simulink library "ESTS_VHSO"  (R2024b)
settings: Solver=VariableStepAuto  StartTime=0.0  StopTime=10.0  RelTol=1e-3
undefined symbols (not defined in the file or in its folder): ESTS_HVSO_p_SwtRefSped_na, p_RatGearFr_na, p_RatGearRe_na
libraries: ESTS_BRK x1, ESTS_LNGSL x1, ESTS_RBA x1, ESTS_REV x1, ESTS_RSL x1, ESTS_SLA x1, ESTS_TFX x1, ESTS_VSLARE x1, ESTS_TFY x1
settings Model: Creator=blatak  LastModifiedBy=blatak
settings ModelReferenceCC: EnableRefExpFcnMdlSchedulingChecks=on
settings RTWCC: GPUComputeCapability=3.5

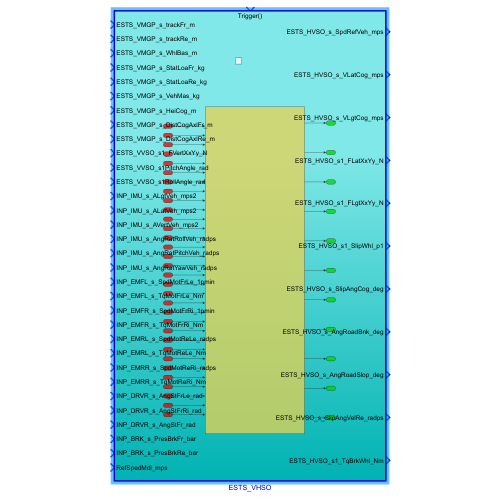
[thumbnail: Simulink's stored preview of the top-level diagram]
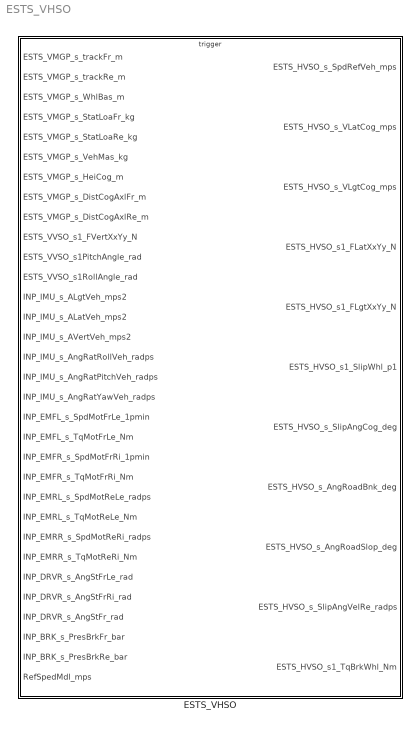
== system ESTS_VHSO ==
  ESTS_VHSO : Subsystem  Description=Horizontal vehicle observer

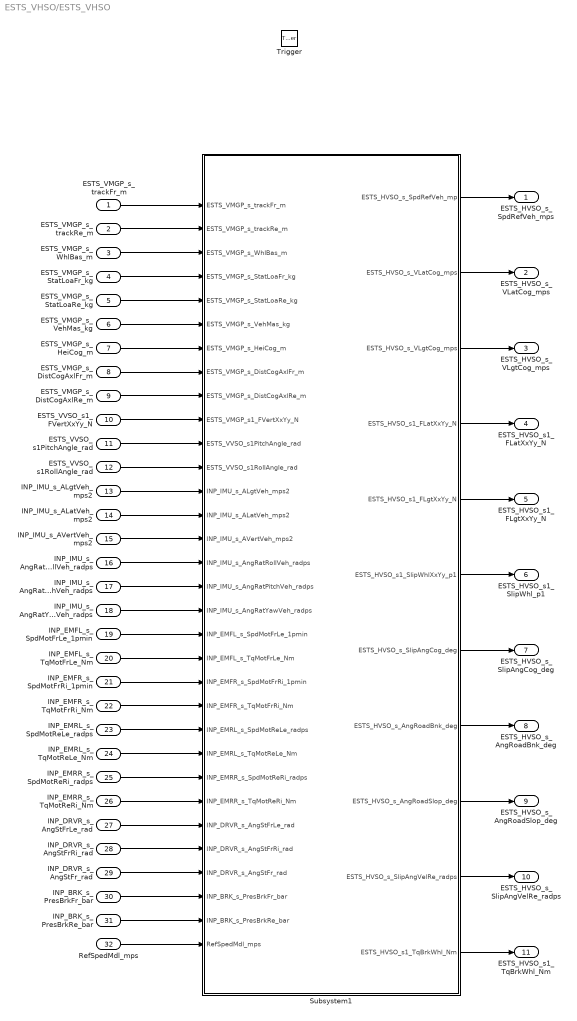
== system ESTS_VHSO/ESTS_VHSO ==
  ESTS_VMGP_s_trackFr_m : Inport
  ESTS_VMGP_s_trackRe_m : Inport  Port=2
  ESTS_VMGP_s_WhlBas_m : Inport  Port=3
  ESTS_VMGP_s_StatLoaFr_kg : Inport  Port=4
  ESTS_VMGP_s_StatLoaRe_kg : Inport  Port=5
  ESTS_VMGP_s_VehMas_kg : Inport  Port=6
  ESTS_VMGP_s_HeiCog_m : Inport  Port=7
  ESTS_VMGP_s_DistCogAxlFr_m : Inport  Port=8
  ESTS_VMGP_s_DistCogAxlRe_m : Inport  Port=9
  ESTS_VVSO_s1_FVertXxYy_N : Inport  Port=10
  ESTS_VVSO_s1PitchAngle_rad : Inport  Port=11
  ESTS_VVSO_s1RollAngle_rad : Inport  Port=12
  INP_IMU_s_ALgtVeh_mps2 : Inport  Port=13
  INP_IMU_s_ALatVeh_mps2 : Inport  Port=14
  INP_IMU_s_AVertVeh_mps2 : Inport  Port=15
  INP_IMU_s_AngRatRollVeh_radps : Inport  Port=16
  INP_IMU_s_AngRatPitchVeh_radps : Inport  Port=17
  INP_IMU_s_AngRatYawVeh_radps : Inport  Port=18
  INP_EMFL_s_SpdMotFrLe_1pmin : Inport  Port=19
  INP_EMFL_s_TqMotFrLe_Nm : Inport  Port=20
  INP_EMFR_s_SpdMotFrRi_1pmin : Inport  Port=21
  INP_EMFR_s_TqMotFrRi_Nm : Inport  Port=22
  INP_EMRL_s_SpdMotReLe_radps : Inport  Port=23
  INP_EMRL_s_TqMotReLe_Nm : Inport  Port=24
  INP_EMRR_s_SpdMotReRi_radps : Inport  Port=25
  INP_EMRR_s_TqMotReRi_Nm : Inport  Port=26
  INP_DRVR_s_AngStFrLe_rad : Inport  Port=27
  INP_DRVR_s_AngStFrRi_rad : Inport  Port=28
  INP_DRVR_s_AngStFr_rad : Inport  Port=29
  INP_BRK_s_PresBrkFr_bar : Inport  Port=30
  INP_BRK_s_PresBrkRe_bar : Inport  Port=31
  RefSpedMdl_mps : Inport  Port=32
  Trigger : TriggerPort  TriggerType=function-call  VariantControl=(inherit)  PortDimensions=1
  Subsystem1 : Subsystem
  ESTS_HVSO_s_SpdRefVeh_mps : Outport
  ESTS_HVSO_s_VLatCog_mps : Outport  Port=2
  ESTS_HVSO_s_VLgtCog_mps : Outport  Port=3
  ESTS_HVSO_s1_FLatXxYy_N : Outport  Port=4
  ESTS_HVSO_s1_FLgtXxYy_N : Outport  Port=5
  ESTS_HVSO_s1_SlipWhl_p1 : Outport  Port=6
  ESTS_HVSO_s_SlipAngCog_deg : Outport  Port=7
  ESTS_HVSO_s_AngRoadBnk_deg : Outport  Port=8
  ESTS_HVSO_s_AngRoadSlop_deg : Outport  Port=9
  ESTS_HVSO_s_SlipAngVelRe_radps : Outport  Port=10
  ESTS_HVSO_s1_TqBrkWhl_Nm : Outport  Port=11
  wires:
  ESTS_VMGP_s_StatLoaFr_kg/1 -> Subsystem1/4(ESTS_VMGP_s_StatLoaFr_kg)
  ESTS_VMGP_s_WhlBas_m/1 -> Subsystem1/3(ESTS_VMGP_s_WhlBas_m)
  ESTS_VMGP_s_trackRe_m/1 -> Subsystem1/2(ESTS_VMGP_s_trackRe_m)
  ESTS_VMGP_s_trackFr_m/1 -> Subsystem1/1(ESTS_VMGP_s_trackFr_m)
  Subsystem1/1(ESTS_HVSO_s_SpdRefVeh_mp) -> ESTS_HVSO_s_SpdRefVeh_mps/1
  Subsystem1/2(ESTS_HVSO_s_VLatCog_mps) -> ESTS_HVSO_s_VLatCog_mps/1
  Subsystem1/3(ESTS_HVSO_s_VLgtCog_mps) -> ESTS_HVSO_s_VLgtCog_mps/1
  Subsystem1/4(ESTS_HVSO_s1_FLatXxYy_N) -> ESTS_HVSO_s1_FLatXxYy_N/1
  Subsystem1/5(ESTS_HVSO_s1_FLgtXxYy_N) -> ESTS_HVSO_s1_FLgtXxYy_N/1
  Subsystem1/6(ESTS_HVSO_s1_SlipWhlXxYy_p1) -> ESTS_HVSO_s1_SlipWhl_p1/1
  Subsystem1/7(ESTS_HVSO_s_SlipAngCog_deg) -> ESTS_HVSO_s_SlipAngCog_deg/1
  Subsystem1/8(ESTS_HVSO_s_AngRoadBnk_deg) -> ESTS_HVSO_s_AngRoadBnk_deg/1
  Subsystem1/9(ESTS_HVSO_s_AngRoadSlop_deg) -> ESTS_HVSO_s_AngRoadSlop_deg/1
  ESTS_VMGP_s_StatLoaRe_kg/1 -> Subsystem1/5(ESTS_VMGP_s_StatLoaRe_kg)
  ESTS_VMGP_s_VehMas_kg/1 -> Subsystem1/6(ESTS_VMGP_s_VehMas_kg)
  ESTS_VMGP_s_HeiCog_m/1 -> Subsystem1/7(ESTS_VMGP_s_HeiCog_m)
  ESTS_VVSO_s1_FVertXxYy_N/1 -> Subsystem1/10(ESTS_VMGP_s1_FVertXxYy_N)
  ESTS_VVSO_s1PitchAngle_rad/1 -> Subsystem1/11(ESTS_VVSO_s1PitchAngle_rad)
  ESTS_VVSO_s1RollAngle_rad/1 -> Subsystem1/12(ESTS_VVSO_s1RollAngle_rad)
  INP_IMU_s_ALgtVeh_mps2/1 -> Subsystem1/13(INP_IMU_s_ALgtVeh_mps2)
  INP_IMU_s_AngRatYawVeh_radps/1 -> Subsystem1/18(INP_IMU_s_AngRatYawVeh_radps)
  INP_IMU_s_AngRatPitchVeh_radps/1 -> Subsystem1/17(INP_IMU_s_AngRatPitchVeh_radps)
  INP_IMU_s_AngRatRollVeh_radps/1 -> Subsystem1/16(INP_IMU_s_AngRatRollVeh_radps)
  INP_IMU_s_AVertVeh_mps2/1 -> Subsystem1/15(INP_IMU_s_AVertVeh_mps2)
  INP_IMU_s_ALatVeh_mps2/1 -> Subsystem1/14(INP_IMU_s_ALatVeh_mps2)
  Subsystem1/10(ESTS_HVSO_s_SlipAngVelRe_radps) -> ESTS_HVSO_s_SlipAngVelRe_radps/1
  INP_EMFL_s_SpdMotFrLe_1pmin/1 -> Subsystem1/19(INP_EMFL_s_SpdMotFrLe_1pmin)
  INP_EMFL_s_TqMotFrLe_Nm/1 -> Subsystem1/20(INP_EMFL_s_TqMotFrLe_Nm)
  INP_EMFR_s_SpdMotFrRi_1pmin/1 -> Subsystem1/21(INP_EMFR_s_SpdMotFrRi_1pmin)
  INP_EMFR_s_TqMotFrRi_Nm/1 -> Subsystem1/22(INP_EMFR_s_TqMotFrRi_Nm)
  INP_EMRL_s_SpdMotReLe_radps/1 -> Subsystem1/23(INP_EMRL_s_SpdMotReLe_radps)
  INP_EMRL_s_TqMotReLe_Nm/1 -> Subsystem1/24(INP_EMRL_s_TqMotReLe_Nm)
  INP_EMRR_s_SpdMotReRi_radps/1 -> Subsystem1/25(INP_EMRR_s_SpdMotReRi_radps)
  INP_EMRR_s_TqMotReRi_Nm/1 -> Subsystem1/26(INP_EMRR_s_TqMotReRi_Nm)
  ESTS_VMGP_s_DistCogAxlFr_m/1 -> Subsystem1/8(ESTS_VMGP_s_DistCogAxlFr_m)
  ESTS_VMGP_s_DistCogAxlRe_m/1 -> Subsystem1/9(ESTS_VMGP_s_DistCogAxlRe_m)
  INP_DRVR_s_AngStFrLe_rad/1 -> Subsystem1/27(INP_DRVR_s_AngStFrLe_rad)
  INP_DRVR_s_AngStFrRi_rad/1 -> Subsystem1/28(INP_DRVR_s_AngStFrRi_rad)
  INP_DRVR_s_AngStFr_rad/1 -> Subsystem1/29(INP_DRVR_s_AngStFr_rad)
  RefSpedMdl_mps/1 -> Subsystem1/32(RefSpedMdl_mps)
  INP_BRK_s_PresBrkFr_bar/1 -> Subsystem1/30(INP_BRK_s_PresBrkFr_bar)
  INP_BRK_s_PresBrkRe_bar/1 -> Subsystem1/31(INP_BRK_s_PresBrkRe_bar)
  Subsystem1/11(ESTS_HVSO_s1_TqBrkWhl_Nm) -> ESTS_HVSO_s1_TqBrkWhl_Nm/1

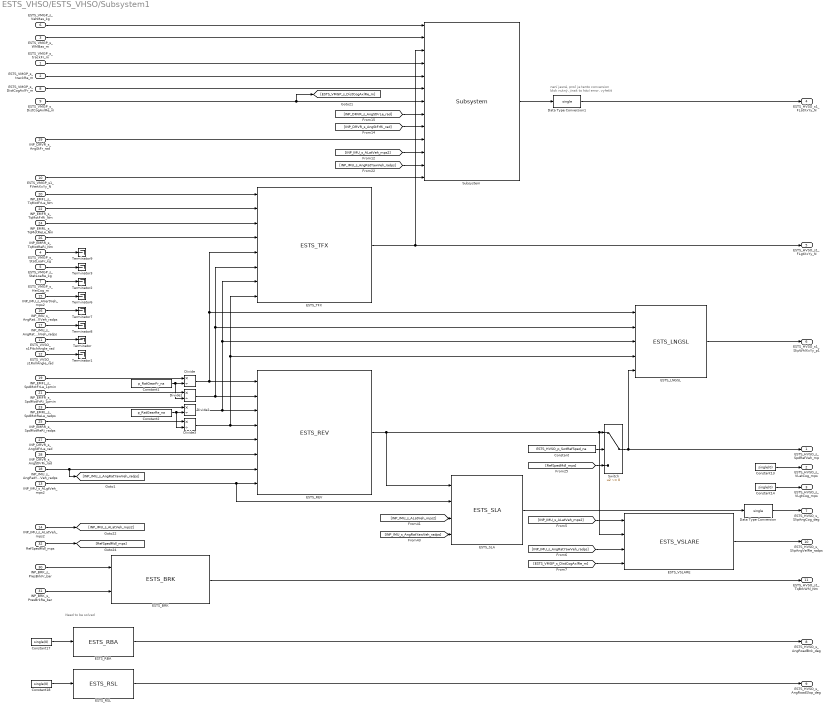
== system ESTS_VHSO/ESTS_VHSO/Subsystem1 ==
  note: není jasné, proč je tento conversion
      | blok nutný, jinak to hází error, vyřešit
  note: Need to be solved
  ESTS_VMGP_s_trackFr_m : Inport
  ESTS_VMGP_s_trackRe_m : Inport  Port=2
  ESTS_VMGP_s_WhlBas_m : Inport  Port=3
  ESTS_VMGP_s_StatLoaFr_kg : Inport  Port=4
  ESTS_VMGP_s_StatLoaRe_kg : Inport  Port=5
  ESTS_VMGP_s_VehMas_kg : Inport  Port=6
  ESTS_VMGP_s_HeiCog_m : Inport  Port=7
  ESTS_VMGP_s_DistCogAxlFr_m : Inport  Port=8
  ESTS_VMGP_s_DistCogAxlRe_m : Inport  Port=9
  ESTS_VMGP_s1_FVertXxYy_N : Inport  Port=10
  ESTS_VVSO_s1PitchAngle_rad : Inport  Port=11
  ESTS_VVSO_s1RollAngle_rad : Inport  Port=12
  INP_IMU_s_ALgtVeh_mps2 : Inport  Port=13
  INP_IMU_s_ALatVeh_mps2 : Inport  Port=14
  INP_IMU_s_AVertVeh_mps2 : Inport  Port=15
  INP_IMU_s_AngRatRollVeh_radps : Inport  Port=16
  INP_IMU_s_AngRatPitchVeh_radps : Inport  Port=17
  INP_IMU_s_AngRatYawVeh_radps : Inport  Port=18
  INP_EMFL_s_SpdMotFrLe_1pmin : Inport  Port=19
  INP_EMFL_s_TqMotFrLe_Nm : Inport  Port=20
  INP_EMFR_s_SpdMotFrRi_1pmin : Inport  Port=21
  INP_EMFR_s_TqMotFrRi_Nm : Inport  Port=22
  INP_EMRL_s_SpdMotReLe_radps : Inport  Port=23
  INP_EMRL_s_TqMotReLe_Nm : Inport  Port=24
  INP_EMRR_s_SpdMotReRi_radps : Inport  Port=25
  INP_EMRR_s_TqMotReRi_Nm : Inport  Port=26
  INP_DRVR_s_AngStFrLe_rad : Inport  Port=27
  INP_DRVR_s_AngStFrRi_rad : Inport  Port=28
  INP_DRVR_s_AngStFr_rad : Inport  Port=29
  INP_BRK_s_PresBrkFr_bar : Inport  Port=30
  INP_BRK_s_PresBrkRe_bar : Inport  Port=31
  RefSpedMdl_mps : Inport  Port=32
  Constant : Constant  Value=ESTS_HVSO_p_SwtRefSped_na
  Constant1 : Constant  Value=p_RatGearFr_na
  Constant{13..14,17..18} (4 alike) : Constant  Value=single(0)
  Constant2 : Constant  Value=p_RatGearRe_na
  Data Type Conversion : DataTypeConversion  OutDataTypeStr=single  SaturateOnIntegerOverflow=off  RndMeth=Floor
  Data Type Conversion1 : DataTypeConversion  OutDataTypeStr=single  SaturateOnIntegerOverflow=off  RndMeth=Floor
  Divide{,1..3} (4 alike) : Product  Inputs=*/
  ESTS_BRK : ESTS_BRK/ESTS_BRK  SystemSampleTime=-1  VariantActivationTime=update diagram  AllowFlexibleInterface=on  Latency=0  AutoFrameSizeCalculation=off
  ESTS_LNGSL : ESTS_LNGSL/ESTS_LNGSL  SystemSampleTime=-1  VariantActivationTime=update diagram  AllowFlexibleInterface=on  Latency=0  AutoFrameSizeCalculation=off
  ESTS_RBA : ESTS_RBA/ESTS_RBA  SystemSampleTime=-1  VariantActivationTime=update diagram  AllowFlexibleInterface=on  Latency=0  AutoFrameSizeCalculation=off
  ESTS_REV : ESTS_REV/ESTS_REV  SystemSampleTime=-1  VariantActivationTime=update diagram  AllowFlexibleInterface=on  Latency=0  AutoFrameSizeCalculation=off
  ESTS_RSL : ESTS_RSL/ESTS_RSL  SystemSampleTime=-1  VariantActivationTime=update diagram  AllowFlexibleInterface=on  Latency=0  AutoFrameSizeCalculation=off
  ESTS_SLA : ESTS_SLA/ESTS_SLA  SystemSampleTime=-1  VariantActivationTime=update diagram  AllowFlexibleInterface=on  Latency=0  AutoFrameSizeCalculation=off
  ESTS_TFX : ESTS_TFX/ESTS_TFX  SystemSampleTime=-1  VariantActivationTime=update diagram  AllowFlexibleInterface=on  Latency=0  AutoFrameSizeCalculation=off
  ESTS_VSLARE : ESTS_VSLARE/ESTS_VSLARE  SystemSampleTime=-1  VariantActivationTime=update diagram  AllowFlexibleInterface=on  Latency=0  AutoFrameSizeCalculation=off
  Subsystem : ESTS_TFY/Subsystem  SystemSampleTime=-1  VariantActivationTime=update diagram  AllowFlexibleInterface=on  Latency=0  AutoFrameSizeCalculation=off
  Switch : Switch  Criteria=u2 ~= 0  SaturateOnIntegerOverflow=off  InputSameDT=off
  Terminator{,1..3,6..9} (8 alike) : Terminator
  ESTS_HVSO_s_SpdRefVeh_mp : Outport
  ESTS_HVSO_s_VLatCog_mps : Outport  Port=2
  ESTS_HVSO_s_VLgtCog_mps : Outport  Port=3
  ESTS_HVSO_s1_FLatXxYy_N : Outport  Port=4
  ESTS_HVSO_s1_FLgtXxYy_N : Outport  Port=5
  ESTS_HVSO_s1_SlipWhlXxYy_p1 : Outport  Port=6
  ESTS_HVSO_s_SlipAngCog_deg : Outport  Port=7
  ESTS_HVSO_s_AngRoadBnk_deg : Outport  Port=8
  ESTS_HVSO_s_AngRoadSlop_deg : Outport  Port=9
  ESTS_HVSO_s_SlipAngVelRe_radps : Outport  Port=10
  ESTS_HVSO_s1_TqBrkWhl_Nm : Outport  Port=11
  wires:
  Constant18/1 -> ESTS_RSL/1
  Constant17/1 -> ESTS_RBA/1
  ESTS_LNGSL/1 -> ESTS_HVSO_s1_SlipWhlXxYy_p1/1
  ESTS_TFX/1 -> Subsystem/3, ESTS_HVSO_s1_FLgtXxYy_N/1
  Constant13/1 -> ESTS_HVSO_s_VLatCog_mps/1
  Constant14/1 -> ESTS_HVSO_s_VLgtCog_mps/1
  ESTS_VSLARE/1 -> ESTS_HVSO_s_SlipAngVelRe_radps/1
  ESTS_RBA/1 -> ESTS_HVSO_s_AngRoadBnk_deg/1
  ESTS_RSL/1 -> ESTS_HVSO_s_AngRoadSlop_deg/1
  INP_EMFL_s_SpdMotFrLe_1pmin/1 -> Divide/1
  INP_EMFR_s_SpdMotFrRi_1pmin/1 -> Divide1/1
  INP_EMFL_s_TqMotFrLe_Nm/1 -> ESTS_TFX/1
  INP_EMRL_s_TqMotReLe_Nm/1 -> ESTS_TFX/3
  INP_EMFR_s_TqMotFrRi_Nm/1 -> ESTS_TFX/2
  INP_EMRR_s_TqMotReRi_Nm/1 -> ESTS_TFX/4
  ESTS_VMGP_s_StatLoaFr_kg/1 -> Terminator9/1
  ESTS_VMGP_s_StatLoaRe_kg/1 -> Terminator3/1
  ESTS_VMGP_s_HeiCog_m/1 -> Terminator2/1
  INP_IMU_s_ALatVeh_mps2/1 -> [INP_IMU_s_ALatVeh_mps2]
  [INP_IMU_s_ALatVeh_mps2] -> Subsystem/11
  ESTS_VMGP_s_WhlBas_m/1 -> Subsystem/2
  ESTS_VMGP_s_VehMas_kg/1 -> Subsystem/1
  ESTS_VMGP_s_trackFr_m/1 -> Subsystem/4
  ESTS_VMGP_s_trackRe_m/1 -> Subsystem/5
  ESTS_VMGP_s_DistCogAxlFr_m/1 -> Subsystem/6
  ESTS_VMGP_s_DistCogAxlRe_m/1 -> Subsystem/7, [ESTS_VMGP_s_DistCogAxlRe_m]
  [INP_DRVR_s_AngStFrLe_rad] -> Subsystem/8
  [INP_DRVR_s_AngStFrRi_rad] -> Subsystem/9
  INP_DRVR_s_AngStFr_rad/1 -> Subsystem/10
  [INP_IMU_s_AngRatYawVeh_radps] -> Subsystem/12
  ESTS_VMGP_s1_FVertXxYy_N/1 -> Subsystem/13
  Subsystem/1 -> Data Type Conversion1/1
  ESTS_REV/1 -> ESTS_VSLARE/2, Switch/1, ESTS_SLA/1
  ESTS_VVSO_s1PitchAngle_rad/1 -> Terminator/1
  ESTS_VVSO_s1RollAngle_rad/1 -> Terminator1/1
  INP_IMU_s_AVertVeh_mps2/1 -> Terminator6/1
  INP_IMU_s_AngRatRollVeh_radps/1 -> Terminator7/1
  INP_IMU_s_AngRatPitchVeh_radps/1 -> Terminator8/1
  RefSpedMdl_mps/1 -> [RefSpedMdl_mps]
  [RefSpedMdl_mps] -> Switch/3
  Switch/1 -> ESTS_HVSO_s_SpdRefVeh_mp/1, ESTS_LNGSL/5
  Constant/1 -> Switch/2
  INP_DRVR_s_AngStFrLe_rad/1 -> ESTS_REV/5
  INP_DRVR_s_AngStFrRi_rad/1 -> ESTS_REV/6
  INP_IMU_s_AngRatYawVeh_radps/1 -> ESTS_REV/7, [INP_IMU_s_AngRatYawVeh_radps]
  ESTS_SLA/1 -> Data Type Conversion/1
  INP_IMU_s_ALgtVeh_mps2/1 -> ESTS_SLA/2, ESTS_REV/8
  [INP_IMU_s_ALatVeh_mps2] -> ESTS_SLA/3
  [INP_IMU_s_AngRatYawVeh_radps] -> ESTS_SLA/4
  [INP_IMU_s_ALatVeh_mps2] -> ESTS_VSLARE/1
  [INP_IMU_s_AngRatYawVeh_radps] -> ESTS_VSLARE/3
  [ESTS_VMGP_s_DistCogAxlRe_m] -> ESTS_VSLARE/4
  Data Type Conversion/1 -> ESTS_HVSO_s_SlipAngCog_deg/1
  Constant1/1 -> Divide1/2, Divide/2
  Divide/1 -> ESTS_LNGSL/1, ESTS_TFX/5, ESTS_REV/1
  Divide1/1 -> ESTS_TFX/6, ESTS_LNGSL/2, ESTS_REV/2
  Divide2/1 -> ESTS_TFX/7, ESTS_LNGSL/3, ESTS_REV/3
  Divide3/1 -> ESTS_TFX/8, ESTS_LNGSL/4, ESTS_REV/4
  Constant2/1 -> Divide3/2, Divide2/2
  INP_EMRL_s_SpdMotReLe_radps/1 -> Divide2/1
  INP_EMRR_s_SpdMotReRi_radps/1 -> Divide3/1
  INP_BRK_s_PresBrkFr_bar/1 -> ESTS_BRK/1
  INP_BRK_s_PresBrkRe_bar/1 -> ESTS_BRK/2
  ESTS_BRK/1 -> ESTS_HVSO_s1_TqBrkWhl_Nm/1
  Data Type Conversion1/1 -> ESTS_HVSO_s1_FLatXxYy_N/1
